simulink model "A310_a"  (R2021b)
settings: Solver=FixedStepDiscrete  StartTime=0.0  StopTime=TSim  RelTol=1e-3
model workspace (MAT data in the model file):
  LengthOfPilot = 16000
undefined symbols (not defined in the file or in its folder): fs, lenPilotSig
libraries: dspsrcs4 x2, dspswit3 x1
settings Model: PacingRate=0.710000  Creator=Feldes  LastModifiedBy=Feldes
settings SolverCC: AlgebraicLoopSolver=TrustRegion  AutoInsertRateTranBlk=on
settings DataIOCC: LimitDataPoints=on  SaveOutput=off  SignalLogging=off  SaveTime=off
settings OptimizationCC: LifeSpan=inf  SimCompilerOptimization=on
settings DebuggingCC: AlgebraicLoopMsg=error  SingleTaskRateTransMsg=error  AllowSymbolicDim=off  SFUnexpectedBacktrackingDiag=warning  SFNoUnconditionalDefaultTransitionDiag=warning  SFExecutionAtInitializationDiag=none  SFMachineParentedDataDiag=warning  ArithmeticOperatorsInVariantConditions=warning
settings SFSimCC: SimUseLocalCustomCode=off  CustomCodeUndefinedFunction=UseInterfaceOnly
settings RTWCC: RTWUseLocalCustomCode=off
settings CodeAppCC: StateflowObjectComments=on
settings GRTTargetCC: TargetLangStandard=C89/C90 (ANSI)
settings ConfigComp: CovMetricSettings=dw  CovSaveCumulativeToWorkspaceVar=on  CovSaveSingleToWorkspaceVar=on  CovExternalEMLEnable=off  CovSFcnEnable=off

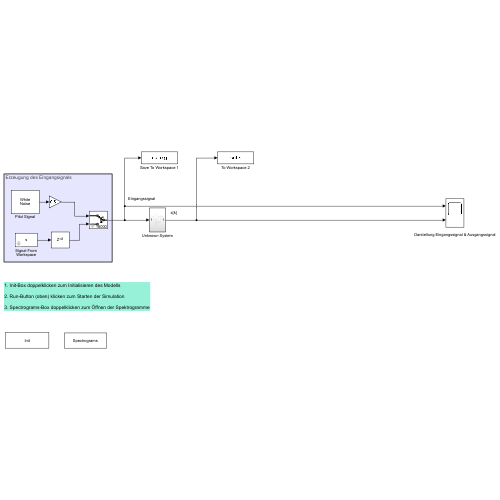
[thumbnail: Simulink's stored preview of the top-level diagram]
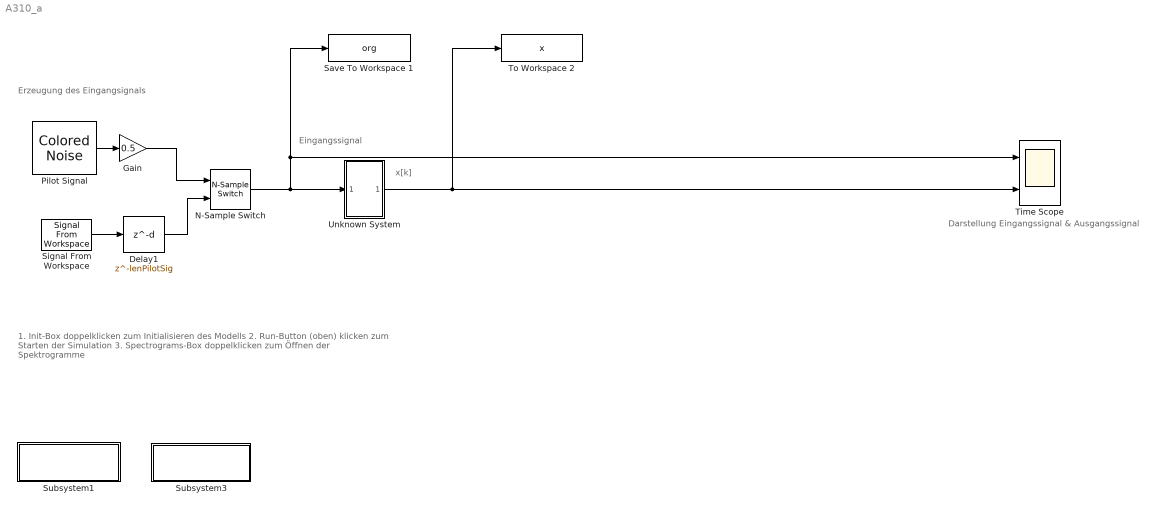
== system A310_a ==
  note: 1. Init-Box doppelklicken zum Initialisieren des Modells
      |
      | 2. Run-Button (oben) klicken zum Starten der Simulation
      |
      | 3. Spectrograms-Box doppelklicken zum Öffnen der Spektrogramme
  note: Erzeugung des Eingangsignals
  note: Darstellung Eingangssignal & Ausgangssignal
  note: x[k]
  note: Eingangssignal
  Delay1 : Delay  DelayLength=lenPilotSig  InputProcessing=Columns as channels (frame based)
  Gain : Gain  Gain=0.5
  N-Sample Switch : dspswit3/N-Sample Switch  N=lenPilotSig  reset=off  TriggerType=Rising edge  Ts=1/fs
      settings: SourceProductBaseCode=DS
  Pilot Signal : dspsrcs4/Colored Noise  Color=white  InverseFrequencyPower=1  BoundedOutput=on  NumChannels=1  OutputDataType=double  SamplesPerFrame=1  SampleTime=1/fs  RandomStream=mt19937ar with seed  Seed=67  SimulateUsing=Interpreted execution
      settings: SourceProductBaseCode=DS
  Save To Workspace 1 : ToWorkspace  VariableName=org  SampleTime=-1
      settings: Save2DSignal=2-D array (concatenate along first dimension)
  Signal From Workspace : dspsrcs4/Signal From Workspace  X=s  Ts=1/fs  nsamps=1  OutputAfterFinalValue=Setting to zero  ignoreOrWarnInputAndFrameLengths=off  OutputFrames=off
  Subsystem1 : Subsystem
      settings: OpenFcn=|
      | lenPilotSig= 16000;
      | [s,fs]=audioread('bbauer8s.wav');
      | TSim =lenPilotSig/fs + length(s)/fs;
      mask Display: disp('Init')
  Subsystem3 : Subsystem
      settings: OpenFcn=|
      | if exist('out','var'), SpectrogramExample(out.org, fs); SpectrogramExample(out.x, fs);
      | else errordlg('You must run the simulation first.','DSP Blockset Demo Error'); end
      mask Display: disp('Spectrograms')
  Time Scope : Scope  NumInputPorts=2
  To Workspace 2 : ToWorkspace  VariableName=x  SampleTime=-1
      settings: Save2DSignal=2-D array (concatenate along first dimension)
  Unknown System : Subsystem
  wires:
  N-Sample Switch/1 -> Save To Workspace 1/1, Time Scope/1, Unknown System/1(In1)
  Unknown System/1(Out1) -> To Workspace 2/1, Time Scope/2
  Pilot Signal/1 -> Gain/1
  Gain/1 -> N-Sample Switch/1
  Signal From Workspace/1 -> Delay1/1
  Delay1/1 -> N-Sample Switch/2

== system A310_a/Subsystem1 ==

== system A310_a/Subsystem3 ==

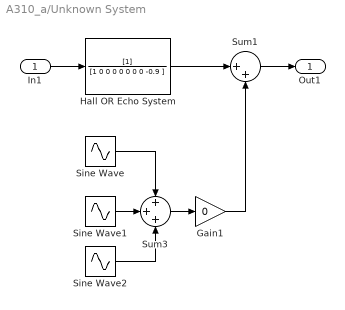
== system A310_a/Unknown System ==
  In1 : Inport
  Gain1 : Gain  Gain=0
  Hall OR Echo System : DiscreteFilter  Denominator=[1 0 0 0 0 0 0 0 -0.9 ]  InputProcessing=Columns as channels (frame based)  FilterStructure=Direct form II transposed  a0EqualsOne=on
  Sine Wave : Sin  Amplitude=1./7.  Frequency=25/40*pi*8000  SampleTime=1/fs
  Sine Wave1 : Sin  Amplitude=1./7.  Frequency=25.1/40*pi*8000  SampleTime=1/fs
  Sine Wave2 : Sin  Amplitude=1./7.  Frequency=25/40*pi*8000  SampleTime=1/fs
  Sum1 : Sum  Inputs=|++  InputSameDT=on  SaturateOnIntegerOverflow=on  OutDataTypeStr=Inherit: Same as first input
  Sum3 : Sum  Inputs=+++  InputSameDT=on  SaturateOnIntegerOverflow=on  OutDataTypeStr=Inherit: Same as first input
  Out1 : Outport
  wires:
  Sum1/1 -> Out1/1
  Hall OR Echo System/1 -> Sum1/1
  Gain1/1 -> Sum1/2
  Sine Wave/1 -> Sum3/1
  Sum3/1 -> Gain1/1
  Sine Wave1/1 -> Sum3/2
  Sine Wave2/1 -> Sum3/3
  In1/1 -> Hall OR Echo System/1
